simulink model "interior_light"  (R2020b)
settings: Solver=VariableStepAuto  StartTime=0.0  StopTime=10  RelTol=1e-3
settings Model: Creator=Training  LastModifiedBy=Training

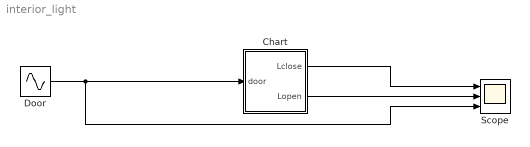
== system interior_light ==
  Chart : Stateflow chart  TreatAsAtomicUnit=on
  "Door " : Sin  Amplitude=5  SampleTime=0
  Scope : Scope  NumInputPorts=3
  wires:
  "Door "/1 -> Chart/1(door), Scope/3
  Chart/1(Lclose) -> Scope/1
  Chart/2(Lopen) -> Scope/2

== stateflow chart interior_light/Chart ==
  state LightOff
    entry:
    statesys=3
    during:
    Lopen=0;
    Lclose=1;
  state LightOn
    entry:
    statesys=1;
    during:
    Lopen=1;
    Lclose=0;
  state BeamReduction
    entry:
    statesys=2;
    during:
    Lclose=0;
    Lopen=door;
  (default) -> LightOn
  BeamReduction -> LightOff [order 2] : [door<=0.5]
  BeamReduction -> LightOn [order 1] : [door>5]
  LightOn -> BeamReduction [order 1] : [door>0.5 && door<=5]
  LightOff -> BeamReduction [order 1] : [door>0.5&& door<=5]
  LightOff -> LightOn [order 2] : [door>5]
  LightOn -> LightOff [order 2] : [door<=0.5]
  data: statesys local; door input; Lclose output; Lopen output
